simulink model "Battery_model_3D_Battery1"  (R2026a)
settings: Solver=VariableStepAuto  StopTime=10000
InitFcn:
  | %% Universal Parameters
  | 
  | Cycle_num = 1000; % number of cycles
  | 
  | Temp_state = 35;
  | Temp = [5, 15, 25, 35, 45];
  | 
  | SoC_state = 0.5;
  | SoC = [0,0.0500000000000000,0.100000000000000,0.150000000000000,0.200000000000000,0.250000000000000,0.300000000000000,0.350000000000000,0.400000000000000,0.450000000000000,0.500000000000000,0.550000000000000,0.600000000000000,0.650000000000000,0.700000000000000,0.750000000000000,0.800000000000000,0.850000000000000,0.900000000000000,0.950000000000000,1];
  | 
  | OCV = [ 3.0025,3.4635,3.521,3.5618,3.6058,3.6426,3.6725,3.7049,3.7486,3.79951,3.8418,3.8738 ,3.9044,3.9448,3.9813,4.0222 ,4.0498,4.0658,4.0919,4.1359,4.2];
  | 
  | % Cn = 540; % As
  | Ru = 3.19; % KW^-1
  | Rc = 1.94; % KW^-1
  | Cc = 62.7; % JK^-1
  | Cs = 4.5;  % JK^-1
  | 
  | Ea = 31500;  % J * mol^-1
  | eta = 152.5; % unitless
  | Ic = 9000;   % [1/s] normalized current rate
  | Rg = 8.314;  % J / K / mol
  | z = 0.57;    % Ah power law exponent
  | 
  | 
  | % Ciclo 175 interpolado (media de ciclos 150 y 200)
  | 
  | Cycle  = [0, 25, 50, 75, 100, 125, 150, 175, 200, 225, 250, 275, 300, 325, 350];
  | SoC    = [0.0, 0.05, 0.1, 0.15, 0.2, 0.25, 0.3, 0.35, 0.4, 0.45, 0.5, 0.55, 0.6, 0.65, 0.7, 0.75, 0.8, 0.85, 0.9, 0.95, 1.0];
  | 
  | % --- R0 ---
  | r0_c0                = [0.14239305, 0.14239305, 0.14239305, 0.12096783, 0.11020203, 0.11749208, 0.15611389, 0.16207555, 0.16172895, 0.16232543, 0.16202235, 0.16165640, 0.16169993, 0.16186275, 0.16221742, 0.16268333, 0.16313795, 0.16298802, 0.16233349, 0.16203041, 0.16121306];
  | r0_c25               = [0.14255010, 0.14255010, 0.14255010, 0.12110125, 0.11032357, 0.11762166, 0.15628607, 0.16225431, 0.16190732, 0.16250446, 0.16220105, 0.16183469, 0.16187827, 0.16204127, 0.16239633, 0.16286275, 0.16331787, 0.16316778, 0.16251253, 0.16220912, 0.16139087];
  | r0_c50               = [0.14258588, 0.14258588, 0.14258588, 0.12113165, 0.11035126, 0.11765119, 0.15632531, 0.16229504, 0.16194796, 0.16254526, 0.16224177, 0.16187532, 0.16191891, 0.16208195, 0.16243710, 0.16290364, 0.16335887, 0.16320874, 0.16255333, 0.16224984, 0.16143138];
  | r0_c75               = [0.14115608, 0.14115608, 0.14115608, 0.11991699, 0.10924470, 0.11647143, 0.15475773, 0.16066760, 0.16032401, 0.16091531, 0.16061486, 0.16025209, 0.16029524, 0.16045665, 0.16080824, 0.16127010, 0.16172077, 0.16157214, 0.16092330, 0.16062286, 0.15981261];
  | r0_c100              = [0.13946724, 0.13946724, 0.13946724, 0.11848226, 0.10793766, 0.11507792, 0.15290616, 0.15874532, 0.15840584, 0.15899007, 0.15869322, 0.15833478, 0.15837741, 0.15853689, 0.15888428, 0.15934061, 0.15978589, 0.15963904, 0.15899796, 0.15870111, 0.15790055];
  | r0_c125              = [0.13890725, 0.13890725, 0.13890725, 0.11800653, 0.10750427, 0.11461586, 0.15229221, 0.15810792, 0.15776980, 0.15835169, 0.15805603, 0.15769903, 0.15774149, 0.15790033, 0.15824632, 0.15870082, 0.15914431, 0.15899805, 0.15835955, 0.15806389, 0.15726655];
  | r0_c150              = [0.14033226, 0.14033226, 0.14033226, 0.11921712, 0.10860712, 0.11579167, 0.15385453, 0.15972990, 0.15938831, 0.15997617, 0.15967747, 0.15931682, 0.15935971, 0.15952018, 0.15986972, 0.16032888, 0.16077692, 0.16062916, 0.15998411, 0.15968542, 0.15887990];
  | r0_c175              = [0.14053160, 0.14053160, 0.14053160, 0.11938646, 0.10876139, 0.11595615, 0.15407307, 0.15995680, 0.15961472, 0.16020341, 0.15990429, 0.15954312, 0.15958608, 0.15974678, 0.16009681, 0.16055662, 0.16100530, 0.16085733, 0.16021136, 0.15991225, 0.15910558];
  | r0_c200              = [0.14073093, 0.14073093, 0.14073093, 0.11955581, 0.10891567, 0.11612063, 0.15429162, 0.16018369, 0.15984112, 0.16043065, 0.16013111, 0.15976943, 0.15981245, 0.15997337, 0.16032390, 0.16078437, 0.16123368, 0.16108550, 0.16043862, 0.16013907, 0.15933126];
  | r0_c225              = [0.14284627, 0.14284627, 0.14284627, 0.12135286, 0.11055279, 0.11786605, 0.15661079, 0.16259142, 0.16224371, 0.16284210, 0.16253805, 0.16217094, 0.16221460, 0.16237795, 0.16273374, 0.16320113, 0.16365720, 0.16350679, 0.16285019, 0.16254614, 0.16172619];
  | r0_c250              = [0.14426401, 0.14426401, 0.14426401, 0.12255728, 0.11165001, 0.11903585, 0.15816513, 0.16420512, 0.16385396, 0.16445829, 0.16415123, 0.16378046, 0.16382456, 0.16398953, 0.16434886, 0.16482088, 0.16528148, 0.16512958, 0.16446645, 0.16415939, 0.16333130];
  | r0_c275              = [0.14386141, 0.14386141, 0.14386141, 0.12221526, 0.11133843, 0.11870366, 0.15772375, 0.16374688, 0.16339670, 0.16399934, 0.16369313, 0.16332341, 0.16336738, 0.16353189, 0.16389021, 0.16436092, 0.16482023, 0.16466876, 0.16400748, 0.16370128, 0.16287550];
  | r0_c300              = [0.14214494, 0.14214494, 0.14214494, 0.12075706, 0.11001001, 0.11728736, 0.15584188, 0.16179315, 0.16144715, 0.16204260, 0.16174004, 0.16137473, 0.16141818, 0.16158072, 0.16193477, 0.16239986, 0.16285369, 0.16270403, 0.16205064, 0.16174809, 0.16093216];
  | r0_c325              = [0.14514692, 0.14514692, 0.14514692, 0.12330734, 0.11233332, 0.11976437, 0.15913312, 0.16521008, 0.16485677, 0.16546479, 0.16515585, 0.16478282, 0.16482719, 0.16499316, 0.16535469, 0.16582960, 0.16629302, 0.16614019, 0.16547301, 0.16516406, 0.16433091];
  | r0_c350              = [0.14384876, 0.14384876, 0.14384876, 0.12220451, 0.11132864, 0.11869322, 0.15770987, 0.16373248, 0.16338233, 0.16398491, 0.16367873, 0.16330904, 0.16335301, 0.16351750, 0.16387580, 0.16434646, 0.16480573, 0.16465427, 0.16399306, 0.16368688, 0.16286117];
  | R0_table = [r0_c0; r0_c25; r0_c50; r0_c75; r0_c100; r0_c125; r0_c150; r0_c175; r0_c200; r0_c225; r0_c250; r0_c275; r0_c300; r0_c325; r0_c350];
  | 
  | % --- R1 ---
  | r1_c0                = [0.05846801, 0.05846801, 0.05947012, 0.04878911, 0.04293380, 0.04603220, 0.06311338, 0.06616573, 0.06571168, 0.06445378, 0.06416472, 0.06367806, 0.06311977, 0.06294519, 0.06280066, 0.06264206, 0.06259538, 0.06286972, 0.06311785, 0.06345615, 0.06395049];
  | r1_c25               = [0.05496513, 0.05496513, 0.05590720, 0.04586610, 0.04036159, 0.04327436, 0.05933219, 0.06220167, 0.06177483, 0.06059228, 0.06032054, 0.05986304, 0.05933820, 0.05917407, 0.05903820, 0.05888911, 0.05884522, 0.05910313, 0.05933639, 0.05965442, 0.06011915];
  | r1_c50               = [0.05573285, 0.05573285, 0.05668808, 0.04650673, 0.04092534, 0.04387879, 0.06016090, 0.06307047, 0.06263766, 0.06143860, 0.06116307, 0.06069917, 0.06016700, 0.06000058, 0.05986281, 0.05971164, 0.05966714, 0.05992865, 0.06016517, 0.06048764, 0.06095886];
  | r1_c75               = [0.05135971, 0.05135971, 0.05223998, 0.04285752, 0.03771408, 0.04043579, 0.05544031, 0.05812157, 0.05772272, 0.05661775, 0.05636384, 0.05593634, 0.05544593, 0.05529257, 0.05516561, 0.05502629, 0.05498529, 0.05522628, 0.05544424, 0.05574141, 0.05617565];
  | r1_c100              = [0.05137385, 0.05137385, 0.05225436, 0.04286932, 0.03772447, 0.04044693, 0.05545557, 0.05813757, 0.05773862, 0.05663334, 0.05637935, 0.05595174, 0.05546119, 0.05530779, 0.05518080, 0.05504144, 0.05500042, 0.05524148, 0.05545951, 0.05575676, 0.05619111];
  | r1_c125              = [0.05125881, 0.05125881, 0.05213735, 0.04277333, 0.03763999, 0.04035635, 0.05533139, 0.05800738, 0.05760932, 0.05650652, 0.05625310, 0.05582645, 0.05533700, 0.05518394, 0.05505723, 0.05491819, 0.05487726, 0.05511778, 0.05533531, 0.05563190, 0.05606528];
  | r1_c150              = [0.06058201, 0.06058201, 0.06162034, 0.05055315, 0.04448613, 0.04769656, 0.06539533, 0.06855805, 0.06808758, 0.06678420, 0.06648469, 0.06598043, 0.06540196, 0.06522106, 0.06507131, 0.06490697, 0.06485860, 0.06514287, 0.06539997, 0.06575050, 0.06626271];
  | r1_c175              = [0.05838600, 0.05838600, 0.05938670, 0.04872067, 0.04287358, 0.04596763, 0.06302485, 0.06607292, 0.06561951, 0.06436337, 0.06407472, 0.06358874, 0.06303123, 0.06285689, 0.06271257, 0.06255419, 0.06250758, 0.06278154, 0.06302932, 0.06336714, 0.06386079];
  | r1_c200              = [0.05619000, 0.05619000, 0.05715306, 0.04688820, 0.04126102, 0.04423870, 0.06065437, 0.06358780, 0.06315144, 0.06194255, 0.06166475, 0.06119705, 0.06066051, 0.06049273, 0.06035383, 0.06020142, 0.06015655, 0.06042021, 0.06065867, 0.06098379, 0.06145886];
  | r1_c225              = [0.05836542, 0.05836542, 0.05936577, 0.04870350, 0.04285847, 0.04595143, 0.06300264, 0.06604964, 0.06559638, 0.06434069, 0.06405214, 0.06356633, 0.06300902, 0.06283474, 0.06269047, 0.06253215, 0.06248555, 0.06275941, 0.06300710, 0.06334481, 0.06383828];
  | r1_c250              = [0.05601070, 0.05601070, 0.05697069, 0.04673858, 0.04112936, 0.04409754, 0.06046083, 0.06338490, 0.06294993, 0.06174489, 0.06146799, 0.06100178, 0.06046695, 0.06029970, 0.06016125, 0.06000932, 0.05996460, 0.06022741, 0.06046511, 0.06078919, 0.06126275];
  | ... (+166 lines)
model workspace (MAT data in the model file):
  C_As = 150
  Cn = 150
  I_c = 1
  I_c_full_charged = 0.0333333333333
  Tc_state = 35.0044118318
  Ts_state = 35.0027406087
  V1_state = 0.00398713164124
  V2_state = 0.00927212980774
  V_cutoff = 3
  V_max = 4.2
  current_SoC = 0.996576803874
undefined symbols (not defined in the file): C1_ch, C1_dis, C2_ch, C2_dis, CycleNumber, R0_ch, R0_dis, R1_ch, R1_dis, R2_ch, R2_dis, V1_ini
libraries: simulink x7
(part 2 of 2)

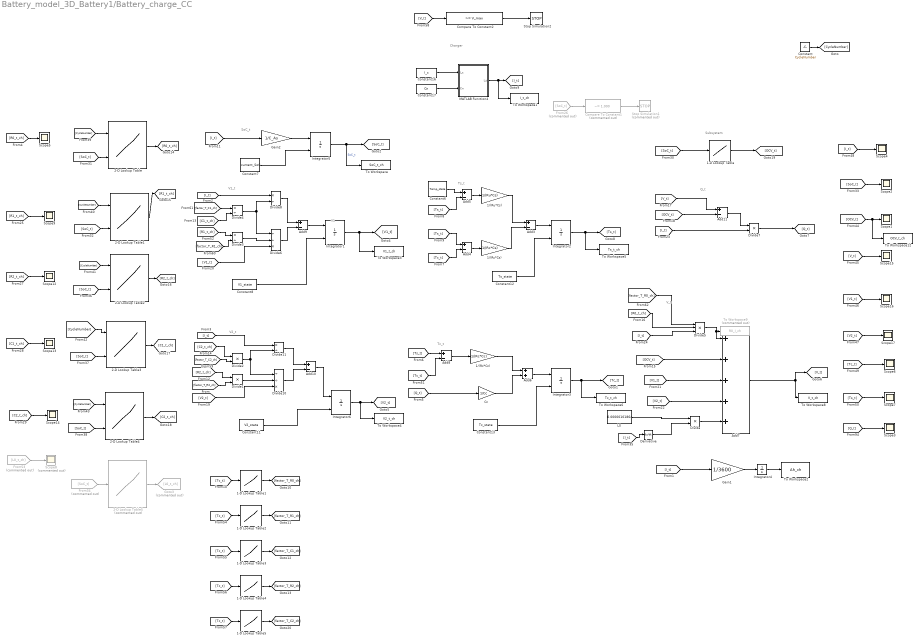
== system Battery_model_3D_Battery1/Battery_charge_CC ==
  note: Subsystem
  note: Tc_t
  note: Ts_t
  note: V_t
  note: V2_t
  note: V1_t
  note: SoC_t
  note: V1
  note: Q_t
  note: Charger
  1-D Lookup Table : Lookup_n-D  NumberOfTableDimensions=1  BreakpointsForDimension1=SoC  BreakpointsForDimension2=Temp  Table=OCV  InternalRulePriority=Speed  RndMeth=Simplest
  1-D Lookup Table1 : Lookup_n-D  NumberOfTableDimensions=1  BreakpointsForDimension1=bp_Tc  Table=factor_T_R0_ch  InternalRulePriority=Speed  RndMeth=Simplest
  1-D Lookup Table2 : Lookup_n-D  NumberOfTableDimensions=1  BreakpointsForDimension1=bp_Tc  Table=factor_T_R1_ch  InternalRulePriority=Speed  RndMeth=Simplest
  1-D Lookup Table3 : Lookup_n-D  NumberOfTableDimensions=1  BreakpointsForDimension1=bp_Tc  Table=factor_T_C1_ch  InternalRulePriority=Speed  RndMeth=Simplest
  1-D Lookup Table4 : Lookup_n-D  NumberOfTableDimensions=1  BreakpointsForDimension1=bp_Tc  Table=factor_T_R2_ch  InternalRulePriority=Speed  RndMeth=Simplest
  1-D Lookup Table5 : Lookup_n-D  NumberOfTableDimensions=1  BreakpointsForDimension1=bp_Tc  Table=factor_T_C2_ch  InternalRulePriority=Speed  RndMeth=Simplest
  1/(Rc*Cc) : Gain  Gain=1/(Rc*Cc)
  1/(Rc*Cs) : Gain  Gain=1/(Rc*Cs)
  1/(Ru*Cs) : Gain  Gain=1/(Ru*Cs)
  2-D Lookup Table : Lookup_n-D  BreakpointsForDimension1=Cycle  BreakpointsForDimension2=SoC  Table=R0_table  InternalRulePriority=Speed  RndMeth=Simplest
      settings: InputPortMap=u0,u1
  2-D Lookup Table1 : Lookup_n-D  BreakpointsForDimension1=Cycle  BreakpointsForDimension2=SoC  Table=R1_table  InternalRulePriority=Speed  RndMeth=Simplest
      settings: InputPortMap=u0,u1
  2-D Lookup Table2 : Lookup_n-D  BreakpointsForDimension1=Cycle  BreakpointsForDimension2=SoC  Table=R2_table  InternalRulePriority=Speed  RndMeth=Simplest
      settings: InputPortMap=u0,u1
  2-D Lookup Table3 : Lookup_n-D  BreakpointsForDimension1=Cycle  BreakpointsForDimension2=SoC  Table=C1_table  InternalRulePriority=Speed  RndMeth=Simplest
      settings: InputPortMap=u0,u1
  2-D Lookup Table4 : Lookup_n-D  BreakpointsForDimension1=Cycle  BreakpointsForDimension2=SoC  Table=C2_table  InternalRulePriority=Speed  RndMeth=Simplest
      settings: InputPortMap=u0,u1
  2-D Lookup Table5 : Lookup_n-D  Commented=on  NumberOfTableDimensions=1  BreakpointsForDimension1=Temp  BreakpointsForDimension2=SoC  Table=C2_ch  InternalRulePriority=Speed  RndMeth=Simplest
  Add{3..5,8..11} (7 alike) : Sum  Inputs=+-
  Add6 : Sum
  Add7 : Sum  Inputs=+++++
  Cc : Gain  Gain=1/Cc
  Compare To Constant1 : simulink/Logic and Bit Operations/Compare To Constant  Commented=on  relop=~=  const=1.000  OutDataTypeStr=boolean
  Compare To Constant2 : simulink/Logic and Bit Operations/Compare To Constant  relop=>=  const=V_max  OutDataTypeStr=boolean
  Constant : Constant  Value=CycleNumber
  Constant11 : Constant  Value=V2_state
  Constant12 : Constant  Value=Ts_state
  Constant13 : Constant  Value=Tc_state
  Constant16 : Constant  Value=I_c
  Constant17 : Constant  Value=Cn
  Constant6 : Constant  Value=Temp_state
  Constant7 : Constant  Value=current_SoC
  Constant8 : Constant  Value=V1_state
  Derivative : Derivative
  Divide{,1..2,7} (4 alike) : Product  Inputs=**
  Divide10 : Product  Inputs=//*
  Divide{3..4,8,11} (4 alike) : Product  Inputs=*/
  Divide5 : Product  Inputs=***
  Divide6 : Product  Inputs=//*
  From26 : From  Commented=on  GotoTag=SoC_t
  From34 : From  Commented=on  GotoTag=SoC_t
  From53 : From  Commented=on  GotoTag=L0_t_ch
  Gain1 : Gain  Gain=1/3600
  Gain2 : Gain  Gain=1/C_As
  Goto3 : Goto  Commented=on  GotoTag=L0_t_ch
  Integrator{1..3,6} (4 alike) : Integrator  InitialConditionSource=external
  Integrator4 : Integrator
  Integrator5 : Integrator  InitialConditionSource=external  InitialCondition=V1_ini
  L0 : Constant  Value=0.00000101864
  MATLAB Function4 : MATLAB Function  TreatAsAtomicUnit=on
  Scope{1..7,9,12..17} (14 alike) : Scope
      Scope1 settings: ActiveDisplayYMinimum=2.2604  ActiveDisplayYMaximum=3.6664  DataLoggingVariableName=ScopeData7
      Scope12 settings: ActiveDisplayYMinimum=0.00751  ActiveDisplayYMaximum=0.04204  DataLoggingVariableName=ScopeData3
      Scope13 settings: ActiveDisplayYMinimum=1446.0874  ActiveDisplayYMaximum=2982.5444  DataLoggingVariableName=ScopeData4
      Scope14 settings: ActiveDisplayYMinimum=14445.3812  ActiveDisplayYMaximum=112360.8817  DataLoggingVariableName=ScopeData5
      Scope15 settings: ActiveDisplayYMinimum=2.15  ActiveDisplayYMaximum=4.15  DataLoggingVariableName=ScopeData8
      Scope16 settings: ActiveDisplayYMinimum=-0.00306  ActiveDisplayYMaximum=0.0275  DataLoggingVariableName=ScopeData9
      Scope17 settings: ActiveDisplayYMinimum=-0.00274  ActiveDisplayYMaximum=0.02463  DataLoggingVariableName=ScopeData10
      Scope2 settings: ActiveDisplayYMinimum=0.0058466  ActiveDisplayYMaximum=0.025847  DataLoggingVariableName=ScopeData6
      Scope3 settings: ActiveDisplayYMinimum=-7.8351  ActiveDisplayYMaximum=6.6118  DataLoggingVariableName=ScopeData14
      Scope4 settings: ActiveDisplayYMinimum=0.049838  ActiveDisplayYMaximum=0.24984  DataLoggingVariableName=ScopeData11
      Scope5 settings: ActiveDisplayYMinimum=0.00753  ActiveDisplayYMaximum=0.01894
      Scope6 settings: ActiveDisplayYMinimum=24.9953  ActiveDisplayYMaximum=44.9953  DataLoggingVariableName=ScopeData12
      Scope7 settings: ActiveDisplayYMinimum=-5.0616  ActiveDisplayYMaximum=45.5546  DataLoggingVariableName=ScopeData13
      Scope9 settings: ActiveDisplayYMinimum=0.00821  ActiveDisplayYMaximum=0.03092  DataLoggingVariableName=ScopeData2
  Scope8 : Scope  Commented=on
      settings: ActiveDisplayYMinimum=14445.3812  ActiveDisplayYMaximum=112360.8817  DataLoggingVariableName=ScopeData24
  Stop Simulation1 : Stop  Commented=on
  Stop Simulation2 : Stop
  To Workspace : ToWorkspace  VariableName=SoC_t_ch  SampleTime=-1
      settings: Save2DSignal=2-D array (concatenate along first dimension)
  To Workspace1 : ToWorkspace  VariableName=I_t_ch  SaveFormat=Timeseries  SampleTime=-1
      settings: Save2DSignal=2-D array (concatenate along first dimension)
  To Workspace12 : ToWorkspace  VariableName=OCV_t_ch  SampleTime=-1
      settings: Save2DSignal=2-D array (concatenate along first dimension)
  To Workspace2 : ToWorkspace  VariableName=Ah_ch  SampleTime=-1
      settings: Save2DSignal=2-D array (concatenate along first dimension)
  To Workspace3 : ToWorkspace  VariableName=V1_t_ch  SampleTime=-1
      settings: Save2DSignal=2-D array (concatenate along first dimension)
  To Workspace4 : ToWorkspace  VariableName=V2_t_ch  SampleTime=-1
      settings: Save2DSignal=2-D array (concatenate along first dimension)
  To Workspace5 : ToWorkspace  VariableName=Ts_t_ch  SampleTime=-1
      settings: Save2DSignal=2-D array (concatenate along first dimension)
  To Workspace6 : ToWorkspace  VariableName=Tc_t_ch  SampleTime=-1
      settings: Save2DSignal=2-D array (concatenate along first dimension)
  To Workspace8 : ToWorkspace  VariableName=V_t_ch  SaveFormat=Timeseries  SampleTime=-1
      settings: Save2DSignal=2-D array (concatenate along first dimension)
  To Workspace9 : ToWorkspace  Commented=on  VariableName=R0_I_ch  SampleTime=-1
      settings: Save2DSignal=2-D array (concatenate along first dimension)
  wires:
  Divide10/1 -> Add10/2
  Add5/1 -> 1/(Ru*Cs)/1
  Add11/1 -> Divide7/1
  [Tc_t] -> Add4/2
  1/(Rc*Cc)/1 -> Add6/1
  [V2_t] -> Add7/4
  Divide5/1 -> Add7/1, To Workspace9/1
  Add4/1 -> 1/(Rc*Cs)/1
  Divide6/1 -> Add9/2
  [I_t] -> Divide11/1
  [CycleNumber] -> 2-D Lookup Table2/1
  Cc/1 -> Add6/2
  [CycleNumber] -> 2-D Lookup Table/1
  Divide7/1 -> [Q_t]
  1-D Lookup Table/1 -> [OCV_t]
  [SoC_t] -> 2-D Lookup Table1/2
  2-D Lookup Table3/1 -> [C1_t_ch]
  [V2_t] -> Scope17/1
  Add9/1 -> Integrator1/1
  2-D Lookup Table/1 -> [R0_t_ch]
  [Ts_t] -> Scope7/1
  [I_t] -> Scope4/1
  [V2_t] -> Divide10/3
  [R1_t_ch] -> Scope9/1
  Add10/1 -> Integrator6/1
  2-D Lookup Table4/1 -> [C2_t_ch]
  [SoC_t] -> 1-D Lookup Table/1
  [R0_t_ch] -> Scope5/1
  [SoC_t] -> 2-D Lookup Table/2
  [R0_t_ch] -> Divide5/2
  [I_t] -> Divide7/2
  [V1_t] -> Scope16/1
  [C2_t_ch] -> Divide2/1
  Add3/1 -> Integrator2/1
  [V_t] -> Add11/1
  [Q_t] -> Scope3/1
  [I_t] -> Divide5/3
  [SoC_t] -> 2-D Lookup Table3/2
  1/(Rc*Cs)/1 -> Add3/2
  [OCV_t] -> To Workspace12/1, Scope1/1
  [C1_t_ch] -> Scope13/1
  [Tc_t] -> Scope6/1
  Divide8/1 -> Add9/1
  [OCV_t] -> Add11/2
  [V1_t] -> Divide6/3
  [Ts_t] -> Add4/1
  [CycleNumber] -> 2-D Lookup Table1/1
  [CycleNumber] -> 2-D Lookup Table3/1
  Gain2/1 -> Integrator5/1
  Add8/1 -> 1/(Rc*Cc)/1
  [R1_t_ch] -> Divide3/1
  [R2_t_ch] -> Scope12/1
  [Q_t] -> Cc/1
  Add6/1 -> Integrator3/1
  [R2_t_ch] -> Divide1/1
  [Ts_t] -> Add8/1
  2-D Lookup Table2/1 -> [R2_t_ch]
  Divide11/1 -> Add10/1
  [C2_t_ch] -> Scope14/1
  Add7/1 -> To Workspace8/1, [V_t]
  [SoC_t] -> 2-D Lookup Table2/2
  Integrator3/1 -> To Workspace6/1, [Tc_t]
  [Ts_t] -> Add5/2
  [Tc_t] -> Add8/2
  [I_t] -> Divide8/1
  Integrator6/1 -> To Workspace4/1, [V2_t]
  Integrator5/1 -> To Workspace/1, [SoC_t]  "SoC_t"
  Integrator1/1 -> To Workspace3/1, [V1_t]
  [SoC_t] -> Scope2/1
  Constant6/1 -> Add5/1
  2-D Lookup Table1/1 -> [R1_t_ch]
  [V_t] -> Scope15/1
  [SoC_t] -> 2-D Lookup Table4/2
  1/(Ru*Cs)/1 -> Add3/1
  [I_t] -> Gain2/1
  [CycleNumber] -> 2-D Lookup Table4/1
  [OCV_t] -> Add7/2
  [V1_t] -> Add7/3
  [I_t] -> Gain1/1
  Integrator4/1 -> To Workspace2/1
  Gain1/1 -> Integrator4/1
  Integrator2/1 -> To Workspace5/1, [Ts_t]
  From26/1 -> Compare To Constant1/1
  Compare To Constant1/1 -> Stop Simulation1/1
  Constant12/1 -> Integrator2/2
  Constant8/1 -> Integrator1/2
  Constant11/1 -> Integrator6/2
  Constant13/1 -> Integrator3/2
  Constant16/1 -> MATLAB Function4/1(I_c)
  Constant17/1 -> MATLAB Function4/2(Cn)
  [V_t] -> Compare To Constant2/1
  Compare To Constant2/1 -> Stop Simulation2/1
  MATLAB Function4/1(I_t) -> To Workspace1/1, [I_t]
  Constant7/1 -> Integrator5/2
  From34/1 -> 2-D Lookup Table5/1
  2-D Lookup Table5/1 -> Goto3/1
  From53/1 -> Scope8/1
  [I_t] -> Derivative/1
  L0/1 -> Divide/1
  Derivative/1 -> Divide/2
  Divide/1 -> Add7/5
  Constant/1 -> [CycleNumber]
  Divide1/1 -> Divide10/2
  Divide2/1 -> Divide11/2, Divide10/1
  [Tc_t] -> 1-D Lookup Table1/1
  1-D Lookup Table1/1 -> [factor_T_R0_ch]
  [Tc_t] -> 1-D Lookup Table2/1
  1-D Lookup Table2/1 -> [factor_T_R1_ch]
  [Tc_t] -> 1-D Lookup Table3/1
  1-D Lookup Table3/1 -> [factor_T_C1_ch]
  [Tc_t] -> 1-D Lookup Table4/1
  1-D Lookup Table4/1 -> [factor_T_R2_ch]
  [Tc_t] -> 1-D Lookup Table5/1
  1-D Lookup Table5/1 -> [factor_T_C2_ch]
  [factor_T_R2_ch] -> Divide1/2
  [factor_T_C2_ch] -> Divide2/2
  [factor_T_R1_ch] -> Divide3/2
  Divide3/1 -> Divide6/2
  Divide4/1 -> Divide6/1, Divide8/2
  [factor_T_C1_ch] -> Divide4/1
  [C1_t_ch] -> Divide4/2
  [factor_T_R0_ch] -> Divide5/1

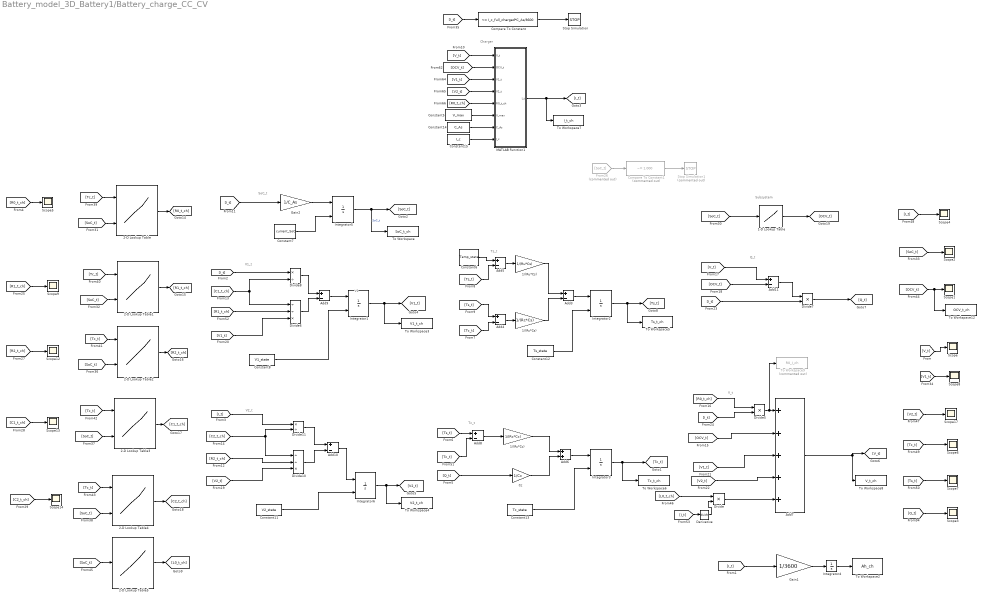
== system Battery_model_3D_Battery1/Battery_charge_CC_CV ==
  note: Subsystem
  note: Tc_t
  note: Ts_t
  note: V_t
  note: V2_t
  note: V1_t
  note: SoC_t
  note: V1
  note: Q_t
  note: Charger
  1-D Lookup Table : Lookup_n-D  NumberOfTableDimensions=1  BreakpointsForDimension1=SoC  BreakpointsForDimension2=Temp  Table=OCV  InternalRulePriority=Speed  RndMeth=Simplest
  1/(Rc*Cc) : Gain  Gain=1/(Rc*Cc)
  1/(Rc*Cs) : Gain  Gain=1/(Rc*Cs)
  1/(Ru*Cs) : Gain  Gain=1/(Ru*Cs)
  2-D Lookup Table : Lookup_n-D  BreakpointsForDimension1=Temp  BreakpointsForDimension2=SoC  Table=R0_ch  InternalRulePriority=Speed  RndMeth=Simplest
      settings: InputPortMap=u0,u1
  2-D Lookup Table1 : Lookup_n-D  BreakpointsForDimension1=Temp  BreakpointsForDimension2=SoC  Table=R1_ch  InternalRulePriority=Speed  RndMeth=Simplest
      settings: InputPortMap=u0,u1
  2-D Lookup Table2 : Lookup_n-D  BreakpointsForDimension1=Temp  BreakpointsForDimension2=SoC  Table=R2_ch  InternalRulePriority=Speed  RndMeth=Simplest
      settings: InputPortMap=u0,u1
  2-D Lookup Table3 : Lookup_n-D  BreakpointsForDimension1=Temp  BreakpointsForDimension2=SoC  Table=C1_ch  InternalRulePriority=Speed  RndMeth=Simplest
      settings: InputPortMap=u0,u1
  2-D Lookup Table4 : Lookup_n-D  BreakpointsForDimension1=Temp  BreakpointsForDimension2=SoC  Table=C2_ch  InternalRulePriority=Speed  RndMeth=Simplest
      settings: InputPortMap=u0,u1
  2-D Lookup Table5 : Lookup_n-D  NumberOfTableDimensions=1  BreakpointsForDimension1=Temp  BreakpointsForDimension2=SoC  Table=C2_ch  InternalRulePriority=Speed  RndMeth=Simplest
  Add{3..5,8..11} (7 alike) : Sum  Inputs=+-
  Add6 : Sum
  Add7 : Sum  Inputs=+++++
  Cc : Gain  Gain=1/Cc
  Compare To Constant : simulink/Logic and Bit Operations/Compare To Constant  relop=<=  const=I_c_full_charged*C_As/3600  OutDataTypeStr=boolean
  Compare To Constant1 : simulink/Logic and Bit Operations/Compare To Constant  Commented=on  relop=~=  const=1.000  OutDataTypeStr=boolean
  Constant11 : Constant  Value=V2_state
  Constant12 : Constant  Value=Ts_state
  Constant13 : Constant  Value=Tc_state
  Constant14 : Constant  Value=C_As
  Constant15 : Constant  Value=I_c
  Constant5 : Constant  Value=V_max
  Constant6 : Constant  Value=Temp_state
  Constant7 : Constant  Value=current_SoC
  Constant8 : Constant  Value=V1_state
  Derivative : Derivative
  Divide : Product  Inputs=**
  Divide10 : Product  Inputs=//*
  Divide11 : Product  Inputs=*/
  Divide5 : Product  Inputs=**
  Divide6 : Product  Inputs=//*
  Divide7 : Product  Inputs=**
  Divide8 : Product  Inputs=*/
  From26 : From  Commented=on  GotoTag=SoC_t
  Gain1 : Gain  Gain=1/3600
  Gain2 : Gain  Gain=1/C_As
  Integrator{1..3,6} (4 alike) : Integrator  InitialConditionSource=external
  Integrator4 : Integrator
  Integrator5 : Integrator  InitialConditionSource=external  InitialCondition=V1_ini
  MATLAB Function1 : MATLAB Function  TreatAsAtomicUnit=on
  Scope{,1..9,12..14,17} (14 alike) : Scope
      Scope settings: ActiveDisplayYMinimum=2.85883  ActiveDisplayYMaximum=4.3268
      Scope1 settings: ActiveDisplayYMinimum=2.85734  ActiveDisplayYMaximum=4.32322  DataLoggingVariableName=ScopeData7
      Scope12 settings: ActiveDisplayYMinimum=0.00751  ActiveDisplayYMaximum=0.04204  DataLoggingVariableName=ScopeData3
      Scope13 settings: ActiveDisplayYMinimum=1446.0874  ActiveDisplayYMaximum=2982.5444  DataLoggingVariableName=ScopeData4
      Scope14 settings: ActiveDisplayYMinimum=14445.3812  ActiveDisplayYMaximum=112360.8817  DataLoggingVariableName=ScopeData5
      Scope17 settings: ActiveDisplayYMinimum=-0.00038  ActiveDisplayYMaximum=0.00342  DataLoggingVariableName=ScopeData10
      Scope2 settings: ActiveDisplayYMinimum=0.00585  ActiveDisplayYMaximum=0.02585  DataLoggingVariableName=ScopeData6
      Scope3 settings: ActiveDisplayYMinimum=-0.00017  ActiveDisplayYMaximum=0.0017  DataLoggingVariableName=ScopeData14
      Scope4 settings: ActiveDisplayYMinimum=0.049838  ActiveDisplayYMaximum=0.24984  DataLoggingVariableName=ScopeData11
      Scope5 settings: ActiveDisplayYMinimum=0.00753  ActiveDisplayYMaximum=0.01894
      Scope6 settings: ActiveDisplayYMinimum=23.74914  ActiveDisplayYMaximum=36.2577  DataLoggingVariableName=ScopeData12
      Scope7 settings: ActiveDisplayYMinimum=23.74954  ActiveDisplayYMaximum=36.2541  DataLoggingVariableName=ScopeData13
      Scope8 settings: DataLoggingVariableName=ScopeData2
      Scope9 settings: ActiveDisplayYMinimum=0.00821  ActiveDisplayYMaximum=0.03092  DataLoggingVariableName=ScopeData2
  Stop Simulation : Stop
  Stop Simulation1 : Stop  Commented=on
  To Workspace : ToWorkspace  VariableName=SoC_t_ch  SampleTime=-1
      settings: Save2DSignal=2-D array (concatenate along first dimension)
  To Workspace12 : ToWorkspace  VariableName=OCV_t_ch  SampleTime=-1
      settings: Save2DSignal=2-D array (concatenate along first dimension)
  To Workspace2 : ToWorkspace  VariableName=Ah_ch  SampleTime=-1
      settings: Save2DSignal=2-D array (concatenate along first dimension)
  To Workspace3 : ToWorkspace  VariableName=V1_t_ch  SampleTime=-1
      settings: Save2DSignal=2-D array (concatenate along first dimension)
  To Workspace4 : ToWorkspace  VariableName=V2_t_ch  SampleTime=-1
      settings: Save2DSignal=2-D array (concatenate along first dimension)
  To Workspace5 : ToWorkspace  VariableName=Ts_t_ch  SampleTime=-1
      settings: Save2DSignal=2-D array (concatenate along first dimension)
  To Workspace6 : ToWorkspace  VariableName=Tc_t_ch  SampleTime=-1
      settings: Save2DSignal=2-D array (concatenate along first dimension)
  To Workspace7 : ToWorkspace  VariableName=I_t_ch  SaveFormat=Timeseries  SampleTime=-1
  To Workspace8 : ToWorkspace  VariableName=V_t_ch  SaveFormat=Timeseries  SampleTime=-1
      settings: Save2DSignal=2-D array (concatenate along first dimension)
  To Workspace9 : ToWorkspace  Commented=on  VariableName=R0_I_ch  SampleTime=-1
      settings: Save2DSignal=2-D array (concatenate along first dimension)
  wires:
  Divide10/1 -> Add10/2
  Add5/1 -> 1/(Ru*Cs)/1
  Add11/1 -> Divide7/1
  [Tc_t] -> Add4/2
  1/(Rc*Cc)/1 -> Add6/1
  [V2_t] -> Add7/4
  Divide5/1 -> To Workspace9/1, Add7/1
  Add4/1 -> 1/(Rc*Cs)/1
  Divide6/1 -> Add9/2
  [I_t] -> Divide11/1
  [Tc_t] -> 2-D Lookup Table2/1
  Cc/1 -> Add6/2
  [Tc_t] -> 2-D Lookup Table/1
  Divide7/1 -> [Q_t]
  1-D Lookup Table/1 -> [OCV_t]
  [SoC_t] -> 2-D Lookup Table1/2
  2-D Lookup Table3/1 -> [C1_t_ch]
  [V2_t] -> Scope17/1
  Add9/1 -> Integrator1/1
  2-D Lookup Table/1 -> [R0_t_ch]
  [Ts_t] -> Scope7/1
  [I_t] -> Scope4/1
  [V2_t] -> Divide10/3
  [R1_t_ch] -> Scope9/1
  Add10/1 -> Integrator6/1
  2-D Lookup Table4/1 -> [C2_t_ch]
  [SoC_t] -> 1-D Lookup Table/1
  [R0_t_ch] -> Scope5/1
  [SoC_t] -> 2-D Lookup Table/2
  [R0_t_ch] -> Divide5/1
  [I_t] -> Divide7/2
  [C2_t_ch] -> Divide10/1, Divide11/2
  Add3/1 -> Integrator2/1
  [V_t] -> Add11/1
  [Q_t] -> Scope3/1
  [I_t] -> Divide5/2
  [SoC_t] -> 2-D Lookup Table3/2
  1/(Rc*Cs)/1 -> Add3/2
  [OCV_t] -> To Workspace12/1, Scope1/1
  [C1_t_ch] -> Scope13/1
  [Tc_t] -> Scope6/1
  Divide8/1 -> Add9/1
  [OCV_t] -> Add11/2
  [V1_t] -> Divide6/3
  [Ts_t] -> Add4/1
  [Tc_t] -> 2-D Lookup Table1/1
  [C1_t_ch] -> Divide8/2, Divide6/1
  [Tc_t] -> 2-D Lookup Table3/1
  Gain2/1 -> Integrator5/1
  Add8/1 -> 1/(Rc*Cc)/1
  [R1_t_ch] -> Divide6/2
  [R2_t_ch] -> Scope12/1
  [Q_t] -> Cc/1
  Add6/1 -> Integrator3/1
  [R2_t_ch] -> Divide10/2
  [Ts_t] -> Add8/1
  2-D Lookup Table2/1 -> [R2_t_ch]
  Divide11/1 -> Add10/1
  [C2_t_ch] -> Scope14/1
  Add7/1 -> [V_t], To Workspace8/1
  [SoC_t] -> 2-D Lookup Table2/2
  Integrator3/1 -> To Workspace6/1, [Tc_t]
  [Ts_t] -> Add5/2
  [Tc_t] -> Add8/2
  [I_t] -> Divide8/1
  Integrator6/1 -> To Workspace4/1, [V2_t]
  Integrator5/1 -> To Workspace/1, [SoC_t]  "SoC_t"
  Integrator1/1 -> To Workspace3/1, [V1_t]
  [SoC_t] -> Scope2/1
  Constant6/1 -> Add5/1
  2-D Lookup Table1/1 -> [R1_t_ch]
  [SoC_t] -> 2-D Lookup Table4/2
  1/(Ru*Cs)/1 -> Add3/1
  [I_t] -> Gain2/1
  [Tc_t] -> 2-D Lookup Table4/1
  [OCV_t] -> Add7/2
  [V1_t] -> Add7/3
  [I_t] -> Gain1/1
  Integrator4/1 -> To Workspace2/1
  Gain1/1 -> Integrator4/1
  Integrator2/1 -> To Workspace5/1, [Ts_t]
  [I_t] -> Compare To Constant/1
  Compare To Constant/1 -> Stop Simulation/1
  [V1_t] -> MATLAB Function1/3(V1_t)
  [R0_t_ch] -> MATLAB Function1/5(R0_t_ch)
  [OCV_t] -> MATLAB Function1/2(OCV_t)
  [V_t] -> MATLAB Function1/1(V_t)
  [V2_t] -> MATLAB Function1/4(V2_t)
  From26/1 -> Compare To Constant1/1
  Compare To Constant1/1 -> Stop Simulation1/1
  Constant12/1 -> Integrator2/2
  Constant8/1 -> Integrator1/2
  Constant11/1 -> Integrator6/2
  Constant13/1 -> Integrator3/2
  Constant14/1 -> MATLAB Function1/7(C_As)
  Constant15/1 -> MATLAB Function1/8(I_c)
  Constant5/1 -> MATLAB Function1/6(V_max)
  MATLAB Function1/1(I_t) -> To Workspace7/1, [I_t]
  Constant7/1 -> Integrator5/2
  [V_t] -> Scope/1
  [V1_t] -> Scope8/1
  [SoC_t] -> 2-D Lookup Table5/1
  2-D Lookup Table5/1 -> [L0_t_ch]
  Derivative/1 -> Divide/2
  [L0_t_ch] -> Divide/1
  [I_t] -> Derivative/1
  Divide/1 -> Add7/5

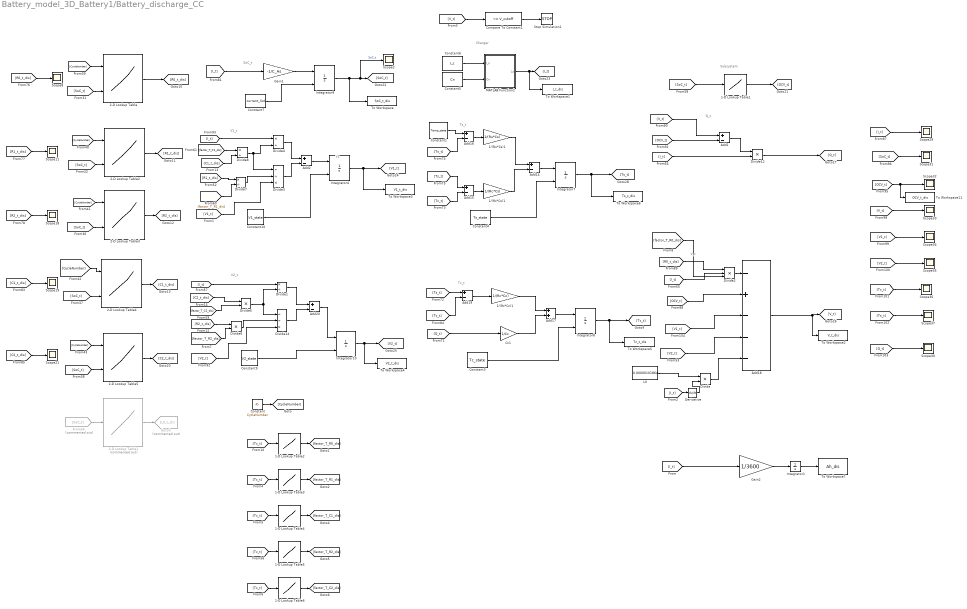
== system Battery_model_3D_Battery1/Battery_discharge_CC ==
  note: Q_t
  note: V1
  note: SoC_t
  note: V1_t
  note: V2_t
  note: V_t
  note: Ts_t
  note: Tc_t
  note: Subsystem
  note: Charger
  1-D Lookup Table1 : Lookup_n-D  NumberOfTableDimensions=1  BreakpointsForDimension1=SoC  BreakpointsForDimension2=Temp  Table=OCV  InternalRulePriority=Speed  RndMeth=Simplest
  1-D Lookup Table2 : Lookup_n-D  NumberOfTableDimensions=1  BreakpointsForDimension1=bp_Tc  Table=factor_T_R0_dis  InternalRulePriority=Speed  RndMeth=Simplest
  1-D Lookup Table3 : Lookup_n-D  NumberOfTableDimensions=1  BreakpointsForDimension1=bp_Tc  Table=factor_T_R1_dis  InternalRulePriority=Speed  RndMeth=Simplest
  1-D Lookup Table4 : Lookup_n-D  NumberOfTableDimensions=1  BreakpointsForDimension1=bp_Tc  Table=factor_T_C1_dis  InternalRulePriority=Speed  RndMeth=Simplest
  1-D Lookup Table5 : Lookup_n-D  NumberOfTableDimensions=1  BreakpointsForDimension1=bp_Tc  Table=factor_T_R2_dis  InternalRulePriority=Speed  RndMeth=Simplest
  1-D Lookup Table6 : Lookup_n-D  NumberOfTableDimensions=1  BreakpointsForDimension1=bp_Tc  Table=factor_T_C2_dis  InternalRulePriority=Speed  RndMeth=Simplest
  1/(Rc*Cc)1 : Gain  Gain=1/(Rc*Cc)
  1/(Rc*Cs)1 : Gain  Gain=1/(Rc*Cs)
  1/(Ru*Cs)1 : Gain  Gain=1/(Ru*Cs)
  2-D Lookup Table : Lookup_n-D  BreakpointsForDimension1=Cycle  BreakpointsForDimension2=SoC  Table=R0_table  InternalRulePriority=Speed  RndMeth=Simplest
      settings: InputPortMap=u0,u1
  2-D Lookup Table1 : Lookup_n-D  Commented=on  NumberOfTableDimensions=1  BreakpointsForDimension1=Temp  BreakpointsForDimension2=SoC  Table=C2_ch  InternalRulePriority=Speed  RndMeth=Simplest
  2-D Lookup Table2 : Lookup_n-D  BreakpointsForDimension1=Cycle  BreakpointsForDimension2=SoC  Table=R1_table  InternalRulePriority=Speed  RndMeth=Simplest
      settings: InputPortMap=u0,u1
  2-D Lookup Table3 : Lookup_n-D  BreakpointsForDimension1=Cycle  BreakpointsForDimension2=SoC  Table=R2_table  InternalRulePriority=Speed  RndMeth=Simplest
      settings: InputPortMap=u0,u1
  2-D Lookup Table4 : Lookup_n-D  BreakpointsForDimension1=Cycle  BreakpointsForDimension2=SoC  Table=C1_table  InternalRulePriority=Speed  RndMeth=Simplest
      settings: InputPortMap=u0,u1
  2-D Lookup Table5 : Lookup_n-D  BreakpointsForDimension1=Cycle  BreakpointsForDimension2=SoC  Table=C2_table  InternalRulePriority=Speed  RndMeth=Simplest
      settings: InputPortMap=u0,u1
  Add{1..2,14..16,19..20} (7 alike) : Sum  Inputs=+-
  Add17 : Sum
  Add18 : Sum  Inputs=-+---
  Cc1 : Gain  Gain=1/Cc
  Compare To Constant1 : simulink/Logic and Bit Operations/Compare To Constant  relop=<=  const=V_cutoff  OutDataTypeStr=boolean
  Constant : Constant  Value=CycleNumber
  Constant1 : Constant  Value=Temp_state
  Constant10 : Constant  Value=V1_state
  Constant3 : Constant  Value=Tc_state
  Constant4 : Constant  Value=Ts_state
  Constant5 : Constant  Value=Cn
  Constant6 : Constant  Value=I_c
  Constant7 : Constant  Value=current_SoC
  Constant9 : Constant  Value=V2_state
  Derivative : Derivative
  Divide{,5..6,12} (4 alike) : Product  Inputs=**
  Divide{1,4,7..8} (4 alike) : Product  Inputs=*/
  Divide14 : Product  Inputs=//*
  Divide2 : Product  Inputs=***
  Divide3 : Product  Inputs=//*
  From34 : From  Commented=on  GotoTag=SoC_t
  Gain1 : Gain  Gain=-1/C_As
  Gain2 : Gain  Gain=1/3600
  Goto3 : Goto  Commented=on  GotoTag=L0_t_ch
  Integrator1 : Integrator
  Integrator{4,7..8,10} (4 alike) : Integrator  InitialConditionSource=external
  Integrator9 : Integrator  InitialConditionSource=external  InitialCondition=V1_ini
  L0 : Constant  Value=0.00000101864
  MATLAB Function2 : MATLAB Function  TreatAsAtomicUnit=on
  Scope{2,8,11,18..19,21,29..37} (15 alike) : Scope
      Scope11 settings: ActiveDisplayYMinimum=-0.125  ActiveDisplayYMaximum=1.125  DataLoggingVariableName=ScopeData7
      Scope18 settings: ActiveDisplayYMinimum=-0.125  ActiveDisplayYMaximum=1.125  DataLoggingVariableName=ScopeData8
      Scope19 settings: ActiveDisplayYMinimum=-0.125  ActiveDisplayYMaximum=1.125  DataLoggingVariableName=ScopeData9
      Scope2 settings: ActiveDisplayYMinimum=-1  ActiveDisplayYMaximum=1
      Scope21 settings: ActiveDisplayYMinimum=-0.125  ActiveDisplayYMaximum=1.125  DataLoggingVariableName=ScopeData10
      Scope29 settings: ActiveDisplayYMinimum=-0.012532  ActiveDisplayYMaximum=0.16806  DataLoggingVariableName=ScopeData15
      Scope30 settings: ActiveDisplayYMinimum=-0.17004  ActiveDisplayYMaximum=1.5304  DataLoggingVariableName=ScopeData23
      Scope31 settings: ActiveDisplayYMinimum=-0.037306  ActiveDisplayYMaximum=0.031954  DataLoggingVariableName=ScopeData16
      Scope32 settings: ActiveDisplayYMinimum=2.8624  ActiveDisplayYMaximum=4.3229  DataLoggingVariableName=ScopeData17
      Scope33 settings: ActiveDisplayYMinimum=2.8623  ActiveDisplayYMaximum=3.1057  DataLoggingVariableName=ScopeData18
      Scope34 settings: ActiveDisplayYMinimum=4.0625E-5  ActiveDisplayYMaximum=0.012439  DataLoggingVariableName=ScopeData19
      Scope35 settings: ActiveDisplayYMinimum=0.00072388  ActiveDisplayYMaximum=0.0085292  DataLoggingVariableName=ScopeData20
      Scope36 settings: ActiveDisplayYMinimum=-4.1824  ActiveDisplayYMaximum=42.6414  DataLoggingVariableName=ScopeData21
      Scope37 settings: ActiveDisplayYMinimum=2.2586  ActiveDisplayYMaximum=3.6824  DataLoggingVariableName=ScopeData22
      Scope8 settings: ActiveDisplayYMinimum=-0.125  ActiveDisplayYMaximum=1.125  DataLoggingVariableName=ScopeData6
  Stop Simulation1 : Stop
  To Workspace : ToWorkspace  VariableName=SoC_t_dis  SampleTime=-1
      settings: Save2DSignal=2-D array (concatenate along first dimension)
  To Workspace1 : ToWorkspace  VariableName=I_t_dis  SaveFormat=Timeseries  SampleTime=-1
  To Workspace11 : ToWorkspace  VariableName=OCV_t_dis  SaveFormat=Timeseries  SampleTime=-1
  To Workspace2 : ToWorkspace  VariableName=V_t_dis  SaveFormat=Timeseries  SampleTime=-1
  To Workspace3 : ToWorkspace  VariableName=V1_t_dis  SampleTime=-1
      settings: Save2DSignal=2-D array (concatenate along first dimension)
  To Workspace4 : ToWorkspace  VariableName=V2_t_dis  SampleTime=-1
      settings: Save2DSignal=2-D array (concatenate along first dimension)
  To Workspace5 : ToWorkspace  VariableName=Tc_t_dis  SampleTime=-1
      settings: Save2DSignal=2-D array (concatenate along first dimension)
  To Workspace6 : ToWorkspace  VariableName=Ts_t_dis  SampleTime=-1
      settings: Save2DSignal=2-D array (concatenate along first dimension)
  To Workspace7 : ToWorkspace  VariableName=Ah_dis  SampleTime=-1
      settings: Save2DSignal=2-D array (concatenate along first dimension)
  wires:
  Add18/1 -> [V_t], To Workspace2/1
  [V2_t] -> Scope35/1
  Cc1/1 -> Add17/2
  Divide1/1 -> Add20/1
  1-D Lookup Table1/1 -> [OCV_t]
  [SoC_t] -> Scope31/1
  Gain1/1 -> Integrator9/1
  [OCV_t] -> Add18/2
  Integrator10/1 -> To Workspace4/1, [V2_t]
  1/(Rc*Cc)1/1 -> Add17/1
  [R0_t_dis] -> Scope8/1
  Integrator4/1 -> To Workspace3/1, [V1_t]
  Divide4/1 -> Add2/1
  [Ts_t] -> Add19/1
  [V2_t] -> Divide14/3
  1/(Ru*Cs)1/1 -> Add14/1
  Add17/1 -> Integrator8/1
  [Tc_t] -> Scope36/1
  Constant1/1 -> Add16/1
  Divide12/1 -> [Q_t]
  Integrator7/1 -> To Workspace6/1, [Ts_t]
  1/(Rc*Cs)1/1 -> Add14/2
  [R1_t_dis] -> Scope11/1
  [Ts_t] -> Add16/2
  [V1_t] -> Add18/3
  Add16/1 -> 1/(Ru*Cs)1/1
  Add1/1 -> Divide12/1
  [I_t] -> Scope29/1
  Divide14/1 -> Add20/2
  [Q_t] -> Scope30/1
  Add14/1 -> Integrator7/1
  Add2/1 -> Integrator4/1
  [V1_t] -> Scope34/1
  2-D Lookup Table3/1 -> [R2_t_dis]
  2-D Lookup Table2/1 -> [R1_t_dis]
  [V2_t] -> Add18/4
  [R2_t_dis] -> Scope18/1
  [OCV_t] -> To Workspace11/1, Scope32/1
  [Q_t] -> Cc1/1
  Divide3/1 -> Add2/2
  [I_t] -> Divide12/2
  Add19/1 -> 1/(Rc*Cc)1/1
  Add20/1 -> Integrator10/1
  [C1_t_dis] -> Scope19/1
  Divide2/1 -> Add18/1
  Add15/1 -> 1/(Rc*Cs)1/1
  Integrator9/1 -> To Workspace/1, Scope2/1, [SoC_t]  "SoC_t"
  [Tc_t] -> Add15/2
  [OCV_t] -> Add1/2
  [C2_t_dis] -> Scope21/1
  [V1_t] -> Divide3/3
  [Ts_t] -> Add15/1
  [Ts_t] -> Scope37/1
  [V_t] -> Scope33/1
  [SoC_t] -> 1-D Lookup Table1/1
  [R0_t_dis] -> Divide2/1
  Integrator8/1 -> To Workspace5/1, [Tc_t]
  [V_t] -> Add1/1
  Constant10/1 -> Integrator4/2
  Constant4/1 -> Integrator7/2
  Constant9/1 -> Integrator10/2
  Constant3/1 -> Integrator8/2
  Integrator1/1 -> To Workspace7/1
  Gain2/1 -> Integrator1/1
  Constant5/1 -> MATLAB Function2/2(Cn)
  Constant6/1 -> MATLAB Function2/1(I_c)
  MATLAB Function2/1(I_t) -> To Workspace1/1, [I_t]
  [V_t] -> Compare To Constant1/1
  Compare To Constant1/1 -> Stop Simulation1/1
  [I_t] -> Gain1/1
  [Tc_t] -> Add19/2
  [I_t] -> Gain2/1
  [I_t] -> Divide4/1
  [I_t] -> Divide1/1
  [I_t] -> Divide2/2
  Constant7/1 -> Integrator9/2
  From34/1 -> 2-D Lookup Table1/1
  2-D Lookup Table1/1 -> Goto3/1
  Derivative/1 -> Divide/2
  Divide/1 -> Add18/5
  [I_t] -> Derivative/1
  L0/1 -> Divide/1
  [CycleNumber] -> 2-D Lookup Table3/1
  2-D Lookup Table4/1 -> [C1_t_dis]
  [CycleNumber] -> 2-D Lookup Table2/1
  [SoC_t] -> 2-D Lookup Table/2
  [CycleNumber] -> 2-D Lookup Table/1
  [SoC_t] -> 2-D Lookup Table2/2
  [SoC_t] -> 2-D Lookup Table3/2
  2-D Lookup Table/1 -> [R0_t_dis]
  [SoC_t] -> 2-D Lookup Table4/2
  [CycleNumber] -> 2-D Lookup Table4/1
  [SoC_t] -> 2-D Lookup Table5/2
  [CycleNumber] -> 2-D Lookup Table5/1
  2-D Lookup Table5/1 -> [C2_t_dis]
  Constant/1 -> [CycleNumber]
  1-D Lookup Table6/1 -> [factor_T_C2_dis]
  [Tc_t] -> 1-D Lookup Table6/1
  [Tc_t] -> 1-D Lookup Table5/1
  [Tc_t] -> 1-D Lookup Table4/1
  [Tc_t] -> 1-D Lookup Table3/1
  1-D Lookup Table4/1 -> [factor_T_C1_dis]
  1-D Lookup Table3/1 -> [factor_T_R1_dis]
  1-D Lookup Table5/1 -> [factor_T_R2_dis]
  [Tc_t] -> 1-D Lookup Table2/1
  1-D Lookup Table2/1 -> [factor_T_R0_dis]
  [R2_t_dis] -> Divide6/1
  [factor_T_R2_dis] -> Divide6/2
  [C2_t_dis] -> Divide5/1
  [factor_T_C2_dis] -> Divide5/2
  Divide6/1 -> Divide14/2
  Divide5/1 -> Divide14/1, Divide1/2
  [factor_T_C1_dis] -> Divide8/1
  [C1_t_dis] -> Divide8/2
  [factor_T_R1_dis] -> Divide7/2
  [R1_t_dis] -> Divide7/1
  Divide8/1 -> Divide3/1, Divide4/2
  Divide7/1 -> Divide3/2
  [factor_T_R0_dis] -> Divide2/3

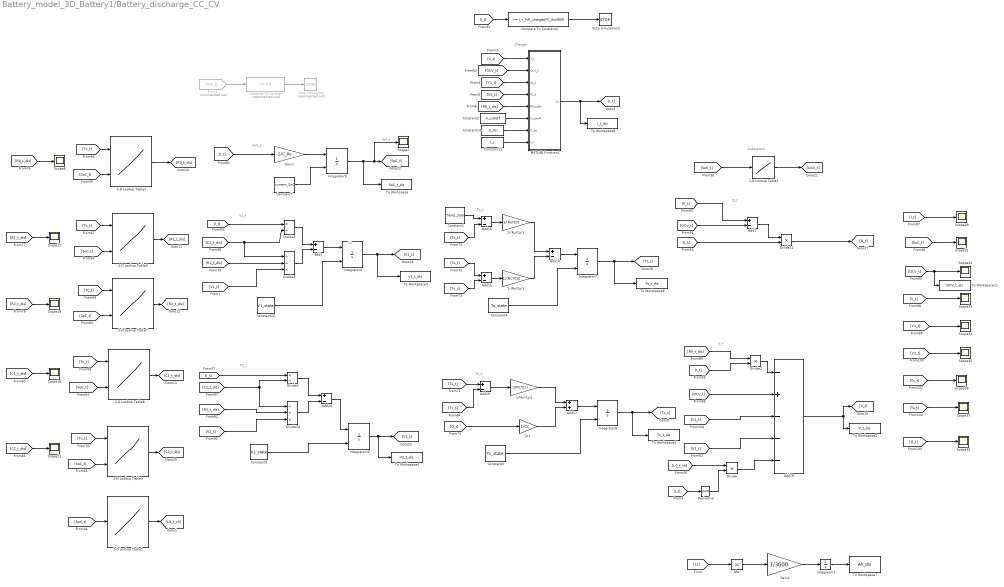
== system Battery_model_3D_Battery1/Battery_discharge_CC_CV ==
  note: Q_t
  note: V1
  note: SoC_t
  note: V1_t
  note: V2_t
  note: V_t
  note: Ts_t
  note: Tc_t
  note: Subsystem
  note: Charger
  1-D Lookup Table1 : Lookup_n-D  NumberOfTableDimensions=1  BreakpointsForDimension1=SoC  BreakpointsForDimension2=Temp  Table=OCV  InternalRulePriority=Speed  RndMeth=Simplest
  1/(Rc*Cc)1 : Gain  Gain=1/(Rc*Cc)
  1/(Rc*Cs)1 : Gain  Gain=1/(Rc*Cs)
  1/(Ru*Cs)1 : Gain  Gain=1/(Ru*Cs)
  2-D Lookup Table1 : Lookup_n-D  NumberOfTableDimensions=1  BreakpointsForDimension1=Temp  BreakpointsForDimension2=SoC  Table=C2_ch  InternalRulePriority=Speed  RndMeth=Simplest
  2-D Lookup Table5 : Lookup_n-D  BreakpointsForDimension1=Temp  BreakpointsForDimension2=SoC  Table=R0_dis  InternalRulePriority=Speed  RndMeth=Simplest
      settings: InputPortMap=u0,u1
  2-D Lookup Table6 : Lookup_n-D  BreakpointsForDimension1=Temp  BreakpointsForDimension2=SoC  Table=R1_dis  InternalRulePriority=Speed  RndMeth=Simplest
      settings: InputPortMap=u0,u1
  2-D Lookup Table7 : Lookup_n-D  BreakpointsForDimension1=Temp  BreakpointsForDimension2=SoC  Table=R2_dis  InternalRulePriority=Speed  RndMeth=Simplest
      settings: InputPortMap=u0,u1
  2-D Lookup Table8 : Lookup_n-D  BreakpointsForDimension1=Temp  BreakpointsForDimension2=SoC  Table=C1_dis  InternalRulePriority=Speed  RndMeth=Simplest
      settings: InputPortMap=u0,u1
  2-D Lookup Table9 : Lookup_n-D  BreakpointsForDimension1=Temp  BreakpointsForDimension2=SoC  Table=C2_dis  InternalRulePriority=Speed  RndMeth=Simplest
      settings: InputPortMap=u0,u1
  Abs : Abs  SaturateOnIntegerOverflow=off
  Add{1..2,14..16,19..20} (7 alike) : Sum  Inputs=+-
  Add17 : Sum
  Add18 : Sum  Inputs=-+---
  Cc1 : Gain  Gain=1/Cc
  Compare To Constant : simulink/Logic and Bit Operations/Compare To Constant  Commented=on  relop=<=  const=0.4  OutDataTypeStr=boolean
  Compare To Constant2 : simulink/Logic and Bit Operations/Compare To Constant  relop=<=  const=I_c_full_charged*C_As/3600  OutDataTypeStr=boolean
  Constant1 : Constant  Value=Temp_state
  Constant10 : Constant  Value=V1_state
  Constant14 : Constant  Value=C_As
  Constant15 : Constant  Value=I_c
  Constant2 : Constant  Value=V_cutoff
  Constant3 : Constant  Value=Tc_state
  Constant4 : Constant  Value=Ts_state
  Constant7 : Constant  Value=current_SoC
  Constant9 : Constant  Value=V2_state
  Derivative : Derivative
  Divide : Product  Inputs=**
  Divide1 : Product  Inputs=*/
  Divide12 : Product  Inputs=**
  Divide14 : Product  Inputs=//*
  Divide2 : Product  Inputs=**
  Divide3 : Product  Inputs=//*
  Divide4 : Product  Inputs=*/
  From2 : From  Commented=on  GotoTag=SoC_t
  Gain1 : Gain  Gain=-1/C_As
  Gain2 : Gain  Gain=1/3600
  Integrator1 : Integrator
  Integrator{4,7..8,10} (4 alike) : Integrator  InitialConditionSource=external
  Integrator9 : Integrator  InitialConditionSource=external  InitialCondition=V1_ini
  MATLAB Function1 : MATLAB Function  TreatAsAtomicUnit=on
  Scope{2,8,11,18..19,21,29..37} (15 alike) : Scope
      Scope11 settings: ActiveDisplayYMinimum=-0.125  ActiveDisplayYMaximum=1.125  DataLoggingVariableName=ScopeData7
      Scope18 settings: ActiveDisplayYMinimum=-0.125  ActiveDisplayYMaximum=1.125  DataLoggingVariableName=ScopeData8
      Scope19 settings: ActiveDisplayYMinimum=-0.125  ActiveDisplayYMaximum=1.125  DataLoggingVariableName=ScopeData9
      Scope2 settings: ActiveDisplayYMinimum=-1  ActiveDisplayYMaximum=1
      Scope21 settings: ActiveDisplayYMinimum=-0.125  ActiveDisplayYMaximum=1.125  DataLoggingVariableName=ScopeData10
      Scope29 settings: ActiveDisplayYMinimum=-0.013121  ActiveDisplayYMaximum=0.16808  DataLoggingVariableName=ScopeData15
      Scope30 settings: ActiveDisplayYMinimum=-0.17004  ActiveDisplayYMaximum=1.5304  DataLoggingVariableName=ScopeData23
      Scope31 settings: ActiveDisplayYMinimum=0.00061627  ActiveDisplayYMaximum=0.00083875  DataLoggingVariableName=ScopeData16
      Scope32 settings: ActiveDisplayYMinimum=2.011  ActiveDisplayYMaximum=4.011  DataLoggingVariableName=ScopeData17
      Scope33 settings: ActiveDisplayYMinimum=2.85  ActiveDisplayYMaximum=3.15  DataLoggingVariableName=ScopeData18
      Scope34 settings: ActiveDisplayYMinimum=0.0016856  ActiveDisplayYMaximum=0.0018374  DataLoggingVariableName=ScopeData19
      Scope35 settings: ActiveDisplayYMinimum=0.006752  ActiveDisplayYMaximum=0.008752  DataLoggingVariableName=ScopeData20
      Scope36 settings: ActiveDisplayYMinimum=-4.1824  ActiveDisplayYMaximum=42.6414  DataLoggingVariableName=ScopeData21
      Scope37 settings: ActiveDisplayYMinimum=2.2586  ActiveDisplayYMaximum=3.6824  DataLoggingVariableName=ScopeData22
      Scope8 settings: ActiveDisplayYMinimum=-0.125  ActiveDisplayYMaximum=1.125  DataLoggingVariableName=ScopeData6
  Stop Simulation : Stop  Commented=on
  Stop Simulation2 : Stop
  To Workspace : ToWorkspace  VariableName=SoC_t_dis  SampleTime=-1
      settings: Save2DSignal=2-D array (concatenate along first dimension)
  To Workspace11 : ToWorkspace  VariableName=OCV_t_dis  SaveFormat=Timeseries  SampleTime=-1
  To Workspace2 : ToWorkspace  VariableName=V_t_dis  SaveFormat=Timeseries  SampleTime=-1
  To Workspace3 : ToWorkspace  VariableName=V1_t_dis  SampleTime=-1
      settings: Save2DSignal=2-D array (concatenate along first dimension)
  To Workspace4 : ToWorkspace  VariableName=V2_t_dis  SampleTime=-1
      settings: Save2DSignal=2-D array (concatenate along first dimension)
  To Workspace5 : ToWorkspace  VariableName=Tc_t_dis  SampleTime=-1
      settings: Save2DSignal=2-D array (concatenate along first dimension)
  To Workspace6 : ToWorkspace  VariableName=Ts_t_dis  SampleTime=-1
      settings: Save2DSignal=2-D array (concatenate along first dimension)
  To Workspace7 : ToWorkspace  VariableName=Ah_dis  SampleTime=-1
      settings: Save2DSignal=2-D array (concatenate along first dimension)
  To Workspace8 : ToWorkspace  VariableName=I_t_dis  SaveFormat=Timeseries  SampleTime=-1
  wires:
  2-D Lookup Table9/1 -> [C2_t_dis]
  [SoC_t] -> 2-D Lookup Table9/2
  Add18/1 -> [V_t], To Workspace2/1
  [V2_t] -> Scope35/1
  Cc1/1 -> Add17/2
  Divide1/1 -> Add20/1
  1-D Lookup Table1/1 -> [OCV_t]
  [SoC_t] -> Scope31/1
  Gain1/1 -> Integrator9/1
  [Tc_t] -> 2-D Lookup Table5/1
  [OCV_t] -> Add18/2
  Integrator10/1 -> To Workspace4/1, [V2_t]
  1/(Rc*Cc)1/1 -> Add17/1
  [R0_t_dis] -> Scope8/1
  Integrator4/1 -> To Workspace3/1, [V1_t]
  Divide4/1 -> Add2/1
  [Ts_t] -> Add19/1
  [C2_t_dis] -> Divide14/1, Divide1/2
  [V2_t] -> Divide14/3
  1/(Ru*Cs)1/1 -> Add14/1
  [SoC_t] -> 2-D Lookup Table8/2
  Add17/1 -> Integrator8/1
  [Tc_t] -> Scope36/1
  Constant1/1 -> Add16/1
  Divide12/1 -> [Q_t]
  2-D Lookup Table8/1 -> [C1_t_dis]
  Integrator7/1 -> To Workspace6/1, [Ts_t]
  1/(Rc*Cs)1/1 -> Add14/2
  [R1_t_dis] -> Scope11/1
  [Ts_t] -> Add16/2
  [V1_t] -> Add18/3
  Add16/1 -> 1/(Ru*Cs)1/1
  Add1/1 -> Divide12/1
  [I_t] -> Scope29/1
  Divide14/1 -> Add20/2
  [R2_t_dis] -> Divide14/2
  [Q_t] -> Scope30/1
  Add14/1 -> Integrator7/1
  Add2/1 -> Integrator4/1
  [Tc_t] -> 2-D Lookup Table7/1
  [V1_t] -> Scope34/1
  2-D Lookup Table7/1 -> [R2_t_dis]
  2-D Lookup Table6/1 -> [R1_t_dis]
  [V2_t] -> Add18/4
  [SoC_t] -> 2-D Lookup Table6/2
  [R2_t_dis] -> Scope18/1
  [SoC_t] -> 2-D Lookup Table5/2
  2-D Lookup Table5/1 -> [R0_t_dis]
  [OCV_t] -> To Workspace11/1, Scope32/1
  [Q_t] -> Cc1/1
  Divide3/1 -> Add2/2
  [I_t] -> Divide12/2
  Add19/1 -> 1/(Rc*Cc)1/1
  Add20/1 -> Integrator10/1
  [C1_t_dis] -> Scope19/1
  Divide2/1 -> Add18/1
  Add15/1 -> 1/(Rc*Cs)1/1
  [R1_t_dis] -> Divide3/2
  [C1_t_dis] -> Divide4/2, Divide3/1
  Integrator9/1 -> To Workspace/1, Scope2/1, [SoC_t]  "SoC_t"
  [Tc_t] -> Add15/2
  [OCV_t] -> Add1/2
  [C2_t_dis] -> Scope21/1
  [Tc_t] -> 2-D Lookup Table8/1
  [V1_t] -> Divide3/3
  [Tc_t] -> 2-D Lookup Table9/1
  [Ts_t] -> Add15/1
  [Ts_t] -> Scope37/1
  [V_t] -> Scope33/1
  [SoC_t] -> 1-D Lookup Table1/1
  [SoC_t] -> 2-D Lookup Table7/2
  [Tc_t] -> 2-D Lookup Table6/1
  [R0_t_dis] -> Divide2/1
  Integrator8/1 -> To Workspace5/1, [Tc_t]
  [V_t] -> Add1/1
  Compare To Constant/1 -> Stop Simulation/1
  From2/1 -> Compare To Constant/1
  Constant10/1 -> Integrator4/2
  Constant4/1 -> Integrator7/2
  Constant9/1 -> Integrator10/2
  Constant3/1 -> Integrator8/2
  [I_t] -> Abs/1
  Integrator1/1 -> To Workspace7/1
  Gain2/1 -> Integrator1/1
  [I_t] -> Gain1/1
  MATLAB Function1/1(I_t) -> To Workspace8/1, [I_t]
  Constant2/1 -> MATLAB Function1/6(V_cutoff)
  Constant14/1 -> MATLAB Function1/7(C_As)
  [R0_t_dis] -> MATLAB Function1/5(R0_t_dis)
  Constant15/1 -> MATLAB Function1/8(I_c)
  [V_t] -> MATLAB Function1/1(V_t)
  [V2_t] -> MATLAB Function1/4(V2_t)
  [OCV_t] -> MATLAB Function1/2(OCV_t)
  [V1_t] -> MATLAB Function1/3(V1_t)
  [Tc_t] -> Add19/2
  [I_t] -> Compare To Constant2/1
  Compare To Constant2/1 -> Stop Simulation2/1
  Abs/1 -> Gain2/1
  [I_t] -> Divide4/1
  [I_t] -> Divide1/1
  [I_t] -> Divide2/2
  Constant7/1 -> Integrator9/2
  [SoC_t] -> 2-D Lookup Table1/1
  2-D Lookup Table1/1 -> [L0_t_ch]
  Derivative/1 -> Divide/2
  Divide/1 -> Add18/5
  [I_t] -> Derivative/1
  [L0_t_ch] -> Divide/1

== matlab function Battery_model_3D_Battery1/Battery_discharge_CC/MATLAB Function2 ==
  data: I_c input; I_t output; Cn input
function I_t = current_control(I_c,Cn)

    I_t = I_c*Cn/3600;
end

== matlab function Battery_model_3D_Battery1/Battery_charge_CC_CV/MATLAB Function1 ==
  data: I_t output; V_t input; OCV_t input; V1_t input; V2_t input; R0_t_ch input; V_max input; C_As input; I_c input
function I_t = current_control(V_t,OCV_t,V1_t,V2_t,R0_t_ch,V_max,C_As,I_c)
   
    if V_t < V_max
        I_t = I_c*C_As/3600;

    else
        I_t = (V_max - OCV_t - V1_t - V2_t)/R0_t_ch;
     
    end    
   
end

== matlab function Battery_model_3D_Battery1/Battery_charge_CC/MATLAB Function4 ==
  data: I_c input; I_t output; Cn input
function I_t = current_control(I_c,Cn)

    I_t = I_c*Cn/3600;
end

== matlab function Battery_model_3D_Battery1/Battery_discharge_CC_CV/MATLAB Function1 ==
  data: I_t output; V_t input; OCV_t input; V1_t input; V2_t input; R0_t_dis input; V_cutoff input; C_As input; I_c input
function I_t = current_control(V_t,OCV_t,V1_t,V2_t,R0_t_dis,V_cutoff,C_As,I_c)
   
    if V_t > V_cutoff
        I_t = I_c*C_As/3600;

    else
        I_t = (-V_cutoff + OCV_t - V1_t - V2_t)/R0_t_dis;
     
    end    
   
end
